simulink model "Ejer11_ContaminantesLagos"  (R2023b)
settings: Solver=VariableStepAuto  StartTime=0.0  StopTime=100  RelTol=1e-3
settings Model: Creator=alfre  LastModifiedBy=alfre

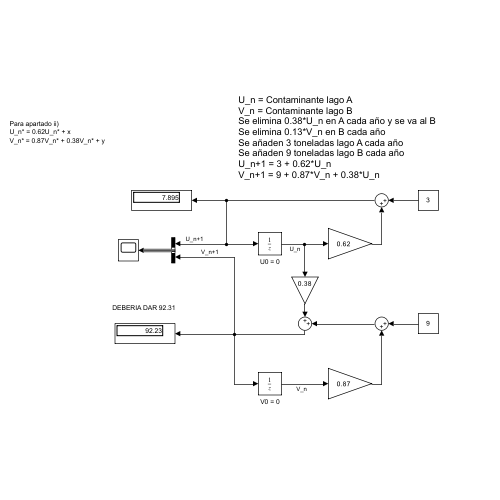
[thumbnail: Simulink's stored preview of the top-level diagram]
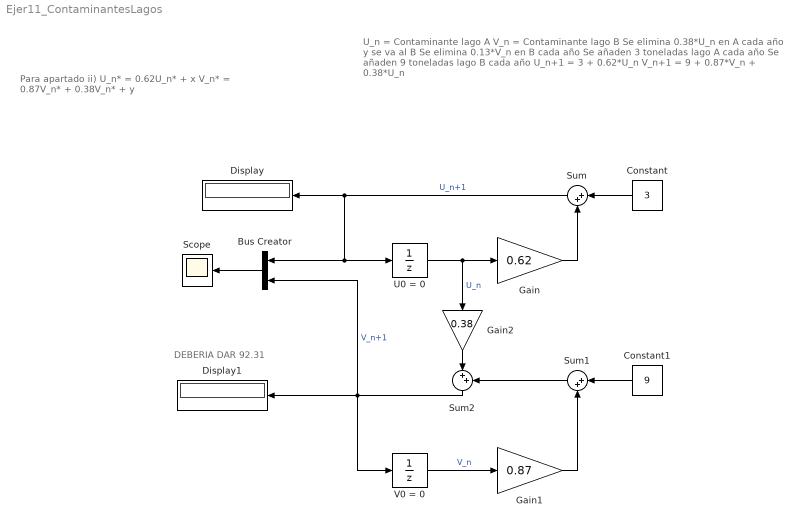
== system Ejer11_ContaminantesLagos ==
  note: Para apartado ii)
      | U_n* = 0.62U_n* + x
      | V_n* = 0.87V_n* + 0.38V_n* + y
  note: DEBERIA DAR 92.31
  note: U_n = Contaminante lago A
      | V_n = Contaminante lago B
      | Se elimina 0.38*U_n en A cada año y se va al B
      | Se elimina 0.13*V_n en B cada año
      | Se añaden 3 toneladas lago A cada año
      | Se añaden 9 toneladas lago B cada año
      | U_n+1 = 3 + 0.62*U_n
      | V_n+1 = 9 + 0.87*V_n + 0.38*U_n
  Bus Creator : BusCreator  Inputs=2
  Constant : Constant  Value=3
  Constant1 : Constant  Value=9
  Display : Display
  Display1 : Display
  Gain : Gain  Gain=0.62
  Gain1 : Gain  Gain=0.87
  Gain2 : Gain  Gain=0.38
  Scope : Scope
  Sum : Sum  Inputs=|++
  Sum1 : Sum  Inputs=|++
  Sum2 : Sum  Inputs=|++
  U0 = 0 : UnitDelay  InitialCondition=3  SampleTime=-1  HasFrameUpgradeWarning=on
  V0 = 0 : UnitDelay  InitialCondition=9  SampleTime=-1  HasFrameUpgradeWarning=on
  wires:
  U0 = 0/1 -> Gain2/1, Gain/1  "U_n"
  Gain/1 -> Sum/2
  Constant/1 -> Sum/1
  Sum/1 -> U0 = 0/1, Bus Creator/1, Display/1  "U_n+1"
  Gain1/1 -> Sum1/2
  V0 = 0/1 -> Gain1/1  "V_n"
  Constant1/1 -> Sum1/1
  Sum1/1 -> Sum2/2
  Sum2/1 -> V0 = 0/1, Display1/1, Bus Creator/2  "V_n+1"
  Bus Creator/1 -> Scope/1
  Gain2/1 -> Sum2/1
